simulink model "vdp2d"  (Simulink 3.00)
settings: Solver=ode45  SolverMode=SingleTasking  StartTime=0.0  StopTime=inf  RelTol=1e-3  AbsTol=1e-6
undefined symbols (not defined in the file or in its folder): sfunxyz
settings Model: ExternalInput=[]  SaveTime=off  SaveOutput=off  InitialState=[]  IntegerOverflowMsg=none  RTWOptions="-aEnforceIntegerDowncast=1 -aFoldNonRolledExpr=1 -aInlineInvariantSignals=1 -aInlineParameters=0 -aLocalBlockOutputs=1 -aRollThreshold=5 -aZeroInternalMemoryAtStartup=1 -aZeroExternalMemoryAtStartup=1 -aInitFltsAndDblsToZero=1 -aGenerateReport=0 -aGenCodeOnly=0 -aRTWVerbose=1 -aIncludeHyperlinkInReport=0 -aLaunchReport=0 -aForceParamTrailComments=0 -aGenerateComments=1 -aIgnoreCustomStorageClasses=1 -aIncHierarchyInIds=0 -aMaxRTWIdLen=31 -aShowEliminatedStatements=0 -aPrefixModelToSubsysFcnNames=1 -aIncDataTypeInIds=0 -aInsertBlockDesc=0 -aSimulinkBlockComments=1 -aInlinedPrmAccess=\"Literals\"  -aSuppressErrorStatus=0 -aModelReferenceCompliant=1 -aSupportNonInlinedSFcns=1 -aSupportContinuousTime=1 -aSupportComplex=1 -aSupportNonFinite=1 -aSupportAbsoluteTime=1 -aTargetFcnLib=\"ansi_tfl_tmw.mat\" -aMultiInstanceERTCode=0 -aLogVarNameModifier=\"rt_\" -aIsPILTarget=0 -aCombineOutputUpdateFcns=0 -aGenerateASAP2=0 -aGenerateSampleERTMain=0 -aGenerateFullHeader=1 -aUtilityFuncGeneration=\"Auto\" -aIncludeFileDelimiter=\"Auto\" -aIncludeMdlTerminateFcn=1 -aPurelyIntegerCode=0 -aERTCustomFileBanners=0 -aRTWCAPIStates=0 -aRTWCAPIParams=0 -aRTWCAPISignals=0 -aMatFileLogging=1 -aGenFloatMathFcnCalls=\"ANSI_C\" -aExtModeMexFile=\"ext_comm\" -aExtModeTransport=0 -aExtModeStaticAllocSize=1000000 -aExtModeTesting=0 -aExtModeStaticAlloc=0 -aExtMode=0  -aInitFltsAndDblsToZero=1 -aInitFltsAndDblsToZero=1"  Creator=The MathWorks Inc.  LastModifiedBy=campa

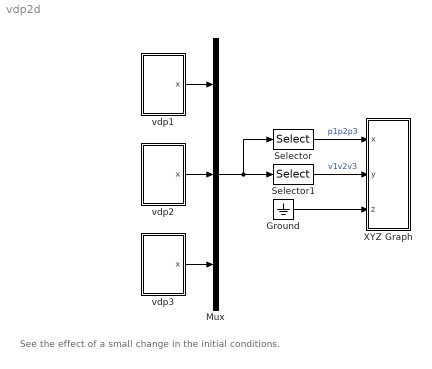
== system vdp2d ==
  note: See the effect of a small change in the initial conditions.
  Ground : Ground
  Mux : Mux  Inputs=[2 2 2]
  Selector : Selector  Elements=[1 3 5]  InputPortWidth=6
  Selector1 : Selector  Elements=[2 4 6]  InputPortWidth=6
  XYZ Graph : Subsystem  LoadFcn=sfunxyz([],[],[],'LoadBlock')  StartFcn=sfunxyz([],[],[],'Start')  StopFcn=sfunxyz([],[],[],'Stop')  mask(XYZ multiscope){np=3, xlim=[-3 3], ylim=[-3 3], zlim=[0 1], cp=[0 0 1], gd=on, st=0.01}
      mask prompts: np "Number of lines"; xlim "[xmin xmax]"; ylim "[ymin ymax]"; zlim "[zmin zmax]"; cp "Camera position (use [0 0 1] for 2D XY view)"; gd "Grid"; st "Sample time:"
      mask help:
      | Multidimensional XYZ scope using MATLAB graph window.
      |    X,Y,Z coordinates are respectively the first,second, and third input.
      |    Enter the number of lines, the XYZ ranges, the camera position,
      |    and the sampling time, as mask parameters.
      settings: CopyFcn=sfunxyz([],[],[],'CopyBlock')  DeleteFcn=sfunxyz([],[],[],'DeleteBlock')  NameChangeFcn=sfunxyz([],[],[],'NameChange')
      mask Help:
      | This block can be used to explore limit cycles.
      |    Look at the m-file sfunxyz.m to see how it works.
      mask Display: plot([.05 .95 .95 .05 .05],[.45 .45 .95 .95 .45], 0.5+cos(0:0.1:2*pi)*0.3,0.7+sin(0:0.1:2*pi)*0.2)
  vdp1 : Subsystem  mask(Van Der Pol System){mu=1, x0=[1 0]}
      mask prompts: x0 "Initial Conditions [p0 v0]"
      mask help: Van Der Pol Oscillator System: xdotdot=mu*xdot*(1-x^2)-x
      mask Help: Van Der Pol Oscillator System: xdotdot=mu*xdot*(1-x^2)-x
  vdp2 : Subsystem  mask(Van Der Pol System){mu=1, x0=[1.5 0]}
      mask prompts: x0 "Initial Conditions [p0 v0]"
      mask help: Van Der Pol Oscillator System: xdotdot=mu*xdot*(1-x^2)-x
      mask Help: Van Der Pol Oscillator System: xdotdot=mu*xdot*(1-x^2)-x
  vdp3 : Subsystem  mask(Van Der Pol System){mu=1, x0=[2.5 0]}
      mask prompts: x0 "Initial Conditions [p0 v0]"
      mask help: Van Der Pol Oscillator System: xdotdot=mu*xdot*(1-x^2)-x
      mask Help: Van Der Pol Oscillator System: xdotdot=mu*xdot*(1-x^2)-x
  wires:
  vdp1/1(x) -> Mux/1
  Mux/1 -> Selector/1, Selector1/1
  Selector/1 -> XYZ Graph/1(x)  "p1p2p3"
  Selector1/1 -> XYZ Graph/2(y)  "v1v2v3"
  Ground/1 -> XYZ Graph/3(z)
  vdp2/1(x) -> Mux/2
  vdp3/1(x) -> Mux/3

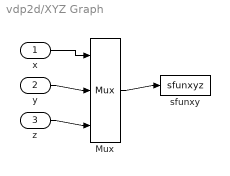
== system vdp2d/XYZ Graph ==
  x : Inport  Port=1  PortWidth=-1  SampleTime=-1  DataType=auto
      settings: SignalType=auto
  y : Inport  Port=2  PortWidth=-1  SampleTime=-1  DataType=auto
      settings: SignalType=auto
  z : Inport  Port=3  PortWidth=-1  SampleTime=-1  DataType=auto
      settings: SignalType=auto
  Mux : Mux  Inputs=[np np np]
      settings: DisplayOption=none
  sfunxy : S-Function  FunctionName=sfunxyz  Parameters=[xlim ylim zlim],st,np,cp,gd  PortCounts=[]  SFunctionModules=''
  wires:
  Mux/1 -> sfunxy/1
  x/1 -> Mux/1
  y/1 -> Mux/2
  z/1 -> Mux/3

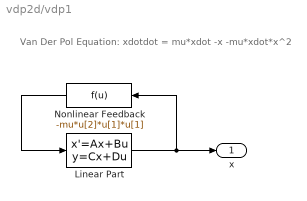
== system vdp2d/vdp1 ==
  note: Van Der Pol Equation: xdotdot = mu*xdot -x -mu*xdot*x^2
  Linear Part : StateSpace  A=[0 1; -1 mu]  B=[0 1]'  C=eye(2)  D=[0 0]'  X0=x0
  Nonlinear Feedback : Fcn  Orientation=left  Expr=-mu*u[2]*u[1]*u[1]
  x : Outport  Port=1
  wires:
  Linear Part/1 -> x/1, Nonlinear Feedback/1
  Nonlinear Feedback/1 -> Linear Part/1

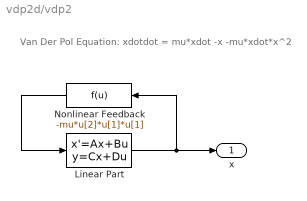
== system vdp2d/vdp2 ==
  note: Van Der Pol Equation: xdotdot = mu*xdot -x -mu*xdot*x^2
  Linear Part : StateSpace  A=[0 1; -1 mu]  B=[0 1]'  C=eye(2)  D=[0 0]'  X0=x0
  Nonlinear Feedback : Fcn  Orientation=left  Expr=-mu*u[2]*u[1]*u[1]
  x : Outport  Port=1
  wires:
  Nonlinear Feedback/1 -> Linear Part/1
  Linear Part/1 -> Nonlinear Feedback/1, x/1

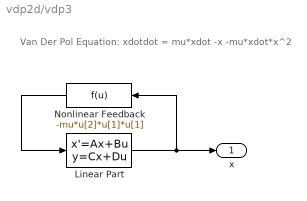
== system vdp2d/vdp3 ==
  note: Van Der Pol Equation: xdotdot = mu*xdot -x -mu*xdot*x^2
  Linear Part : StateSpace  A=[0 1; -1 mu]  B=[0 1]'  C=eye(2)  D=[0 0]'  X0=x0
  Nonlinear Feedback : Fcn  Orientation=left  Expr=-mu*u[2]*u[1]*u[1]
  x : Outport  Port=1
  wires:
  Linear Part/1 -> x/1, Nonlinear Feedback/1
  Nonlinear Feedback/1 -> Linear Part/1
